simulink model "FPGA_Comm_fpu_test1"  (Simulink 7.6)
settings: Solver=FixedStepDiscrete  StartTime=0.0  StopTime=500  FixedStep=0.01  MaxStep=1e-1  RelTol=1e-3
values from neighbouring files (symbols this model uses):
  s2 = op2(1)    [fpu_test.m]
undefined symbols (not defined in the file or in its folder): A_cd, B_cd, C_cd, D_cd
settings Model: Creator=jordan  LastModifiedBy=jordan
settings GRTTargetCC: ExtMode=on

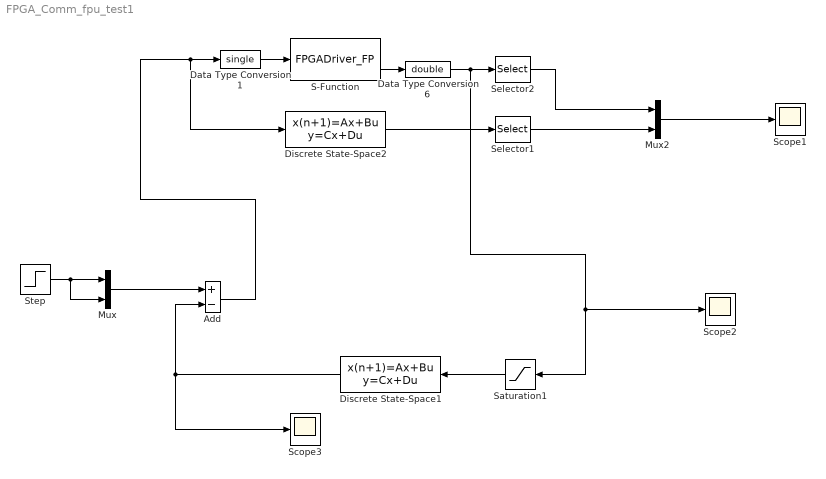
== system FPGA_Comm_fpu_test1 ==
  Add : Sum  Inputs=+-
  Data Type Conversion1 : DataTypeConversion  OutDataTypeStr=single
  Data Type Conversion6 : DataTypeConversion  OutDataTypeStr=double
  Discrete State-Space1 : DiscreteStateSpace  A=s2.a  B=s2.b  C=s2.c  D=s2.d  SampleTime=0.01
  Discrete State-Space2 : DiscreteStateSpace  A=single(A_cd)  B=single(B_cd)  C=single(C_cd)  D=single(D_cd)  SampleTime=0.01
  Mux : Mux  Inputs=2
  Mux2 : Mux  Inputs=2
  S-Function : S-Function  FunctionName=FPGADriver_FP  EnableBusSupport=off
  Saturation1 : Saturate  UpperLimit=5  LowerLimit=-5  LinearizeAsGain=off  RndMeth=Nearest
  Scope1 : Scope
      settings: TimeRange=50  YMin=-115  YMax=0  MaxDataPoints=50000
  Scope2 : Scope
      settings: TimeRange=50  YMin=-10  YMax=170  MaxDataPoints=50000
  Scope3 : Scope
      settings: TimeRange=45  YMin=-0.05  YMax=1.05  SaveName=ScopeData2  MaxDataPoints=50000
  Selector1 : Selector  InputPortWidth=2  IndexOptions=Index vector (dialog)  Indices=2  OutputSizes=1
  Selector2 : Selector  InputPortWidth=2  IndexOptions=Index vector (dialog)  Indices=2  OutputSizes=1
  Step : Step  Time=2
  wires:
  S-Function/2 -> Data Type Conversion6/1
  Data Type Conversion1/1 -> S-Function/1
  Data Type Conversion6/1 -> Selector2/1, Scope2/1, Saturation1/1
  Add/1 -> Data Type Conversion1/1, Discrete State-Space2/1
  Step/1 -> Mux/1, Mux/2
  Mux/1 -> Add/1
  Discrete State-Space1/1 -> Add/2, Scope3/1
  Discrete State-Space2/1 -> Selector1/1
  Mux2/1 -> Scope1/1
  Selector2/1 -> Mux2/1
  Selector1/1 -> Mux2/2
  Saturation1/1 -> Discrete State-Space1/1
